simulink model "Problem9"  (R2020a)
settings: Solver=VariableStepAuto  StartTime=0.0  StopTime=1  RelTol=1e-3
model workspace (MAT data in the model file):
  Ba = 0.01
  Ja = 0.0167
  Kb = 0.8
  Kt = 0.8
  La = 0.003
  Ra = 0.5
  V = 220
settings Model: Creator=tnradm  LastModifiedBy=tnradm

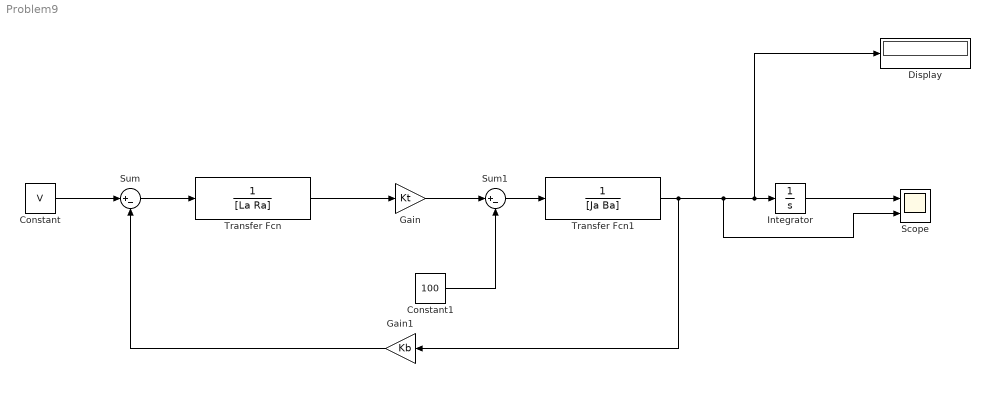
== system Problem9 ==
  Constant : Constant  Value=V
  Constant1 : Constant  Value=100
  Display : Display
  Gain : Gain  Gain=Kt
  Gain1 : Gain  Gain=Kb
  Integrator : Integrator
  Scope : Scope  NumInputPorts=2
  Sum : Sum  Inputs=|+-
  Sum1 : Sum  Inputs=|+-
  Transfer Fcn : TransferFcn  Denominator=[La Ra]
  Transfer Fcn1 : TransferFcn  Denominator=[Ja Ba]
  wires:
  Constant/1 -> Sum/1
  Sum/1 -> Transfer Fcn/1
  Transfer Fcn/1 -> Gain/1
  Gain/1 -> Sum1/1
  Constant1/1 -> Sum1/2
  Integrator/1 -> Scope/1
  Sum1/1 -> Transfer Fcn1/1
  Transfer Fcn1/1 -> Gain1/1, Scope/2, Display/1, Integrator/1
  Gain1/1 -> Sum/2
